simulink model "JGB37_3530_open_loop_motor"  (R2023b)
settings: Solver=ode45  StartTime=0.0  StopTime=5  RelTol=1e-3  EnableMultiTasking=on
settings Model: Creator=yoany  LastModifiedBy=yoany
settings SolverCC: AlgebraicLoopSolver=TrustRegion
settings DataIOCC: LimitDataPoints=on  SaveFormat=Array  SignalLoggingSaveFormat=ModelDataLogs  ReturnWorkspaceOutputs=off
settings OptimizationCC: BooleanDataType=off  LifeSpan=inf
settings DebuggingCC: SaveWithParameterizedLinksMsg=none  UnderspecifiedInitializationDetection=Classic  MergeDetectMultiDrivingBlocksExec=none  SignalResolutionControl=TryResolveAllWithWarning  MultiTaskDSMMsg=warning  MultiTaskCondExecSysMsg=none  UnconnectedInputMsg=warning  UnconnectedOutputMsg=warning  UnconnectedLineMsg=warning  SFUnexpectedBacktrackingDiag=warning  SFNoUnconditionalDefaultTransitionDiag=warning  ArithmeticOperatorsInVariantConditions=warning
settings HardwareCC: TargetUnknown=on
settings ModelReferenceCC: EnableRefExpFcnMdlSchedulingChecks=on  PropagateSignalLabelsOutOfModel=off
settings SFSimCC: SimUseLocalCustomCode=off  CustomCodeUndefinedFunction=UseInterfaceOnly
settings RTWCC: RTWUseLocalCustomCode=off
settings CodeAppCC: StateflowObjectComments=on
settings GRTTargetCC: TargetLangStandard=C89/C90 (ANSI)  CombineOutputUpdateFcns=off  GRTInterface=on
settings ConfigComp: CovMetricSettings=dw  CovSaveCumulativeToWorkspaceVar=on  CovSaveSingleToWorkspaceVar=on  CovExternalEMLEnable=off

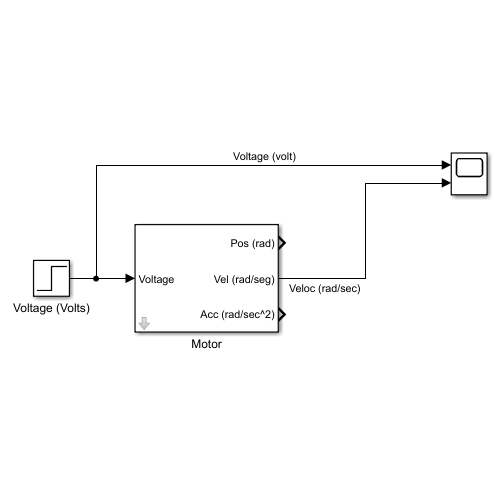
[thumbnail: Simulink's stored preview of the top-level diagram]
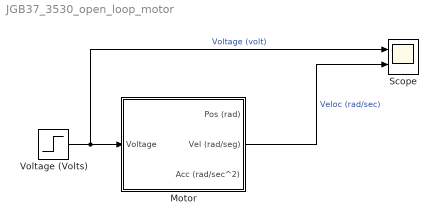
== system JGB37_3530_open_loop_motor ==
  Motor : Subsystem  mask(DC Motor){R=7.5, L=0.5e-3, J=1e-5, b=1e-6, Kt=0.05, Ke=0.05, Re=1/90}
      mask prompts: R "R [Ohm]"; L "L [H]"; J "J [kg.m^2]"; b "b [N.m.s]"; Kt "Kt [N.m/A]"; Ke "Ke [V.s/rad]"
      mask help:
      | Takes the DC voltage as input, and outputs angular position (Pos), velocity (Vel) and acceleration (Acc)
      | R => Equivalent Resistance
      | L  => Equivalent Inductance
      | J   => Moment of Inertia
      | b   => Motor Viscous Friction Constant
      | Kt  => Motor Torque Constant
      | Ke => Electromotive Force Constant
      | Re => Gear Reduction Ratio
  Scope : Scope  NumInputPorts=2
  Voltage (Volts) : Step  After=10  SampleTime=0
  wires:
  Voltage (Volts)/1 -> Scope/1, Motor/1(Voltage)  "Voltage (volt)"
  Motor/2(Vel (rad/seg)) -> Scope/2  "Veloc (rad/sec)"

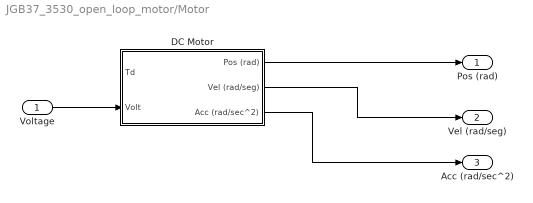
== system JGB37_3530_open_loop_motor/Motor ==
  Voltage : Inport
  "DC Motor " : Subsystem  mask(DC Motor){R=R, L=L, J=J, b=b, Kt=Kt, Ke=Ke, Re=Re}
  Pos (rad) : Outport
  Vel (rad/seg) : Outport  Port=2
  Acc (rad/sec^2) : Outport  Port=3
  wires:
  Voltage/1 -> "DC Motor "/2(Volt)
  "DC Motor "/1(Pos (rad)) -> Pos (rad)/1
  "DC Motor "/2(Vel (rad/seg)) -> Vel (rad/seg)/1
  "DC Motor "/3(Acc (rad/sec^2)) -> Acc (rad/sec^2)/1

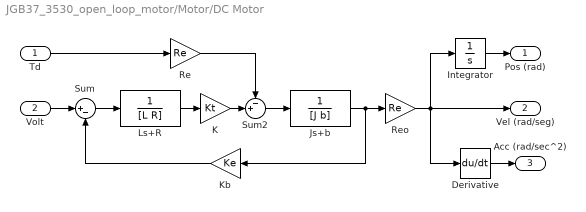
== system JGB37_3530_open_loop_motor/Motor/DC Motor  ==
  Td : Inport
  Volt : Inport  Port=2
  Derivative : Derivative
  Integrator : Integrator
  Js+b : TransferFcn  Denominator=[J b]
  K : Gain  Gain=Kt  SaturateOnIntegerOverflow=on  OutDataTypeStr=Inherit: Same as input  ParamDataTypeStr=Inherit: Same as input
  Kb : Gain  Gain=Ke  SaturateOnIntegerOverflow=on  OutDataTypeStr=Inherit: Same as input  ParamDataTypeStr=Inherit: Same as input
  Ls+R : TransferFcn  Denominator=[L R]
  Re : Gain  Gain=Re  SaturateOnIntegerOverflow=on  OutDataTypeStr=Inherit: Same as input  ParamDataTypeStr=Inherit: Same as input
  Reo : Gain  Gain=Re  SaturateOnIntegerOverflow=on  OutDataTypeStr=Inherit: Same as input  ParamDataTypeStr=Inherit: Same as input
  Sum : Sum  Inputs=|+-  InputSameDT=on  SaturateOnIntegerOverflow=on  OutDataTypeStr=Inherit: Same as first input
  Sum2 : Sum  Inputs=-+|  InputSameDT=on  SaturateOnIntegerOverflow=on  OutDataTypeStr=Inherit: Same as first input
  Pos (rad) : Outport
  Vel (rad/seg) : Outport  Port=2
  Acc (rad/sec^2) : Outport  Port=3
  wires:
  Derivative/1 -> Acc (rad/sec^2)/1
  Integrator/1 -> Pos (rad)/1
  Reo/1 -> Derivative/1, Integrator/1, Vel (rad/seg)/1
  Td/1 -> Re/1
  Volt/1 -> Sum/1
  Re/1 -> Sum2/1
  K/1 -> Sum2/2
  Ls+R/1 -> K/1
  Js+b/1 -> Reo/1, Kb/1
  Sum2/1 -> Js+b/1
  Kb/1 -> Sum/2
  Sum/1 -> Ls+R/1
